simulink model "autopilot2e"  (R2017a)
settings: Solver=VariableStepAuto  StartTime=0.0  StopTime=300  RelTol=1e-3
values from neighbouring files (symbols this model uses):
  a_1 = 2.87    [auoschmilot.m]    (also in run_task_2f.m)
  a_2 = -0.65    [auoschmilot.m]    (also in run_task_2f.m)
  g = 9.81    [auoschmilot.m]    (also in run_task_2f.m)
  k_d_phi = (2*zeta_phi*w_n_phi-a_1)/a_2    [auoschmilot.m]    (also in run_task_2f.m)
  k_i_x = 0.195    [auoschmilot.m]    (also in run_task_2f.m)
  k_p_phi = -5/3    (= -1.66666666667)    [auoschmilot.m]    (also in run_task_2f.m)
  k_p_x = 2*zeta_X*w_n_x*V_g/g    [auoschmilot.m]    (also in run_task_2f.m)
  V_g = 637/3.6    (= 176.944444444)    [auoschmilot.m]    (also in run_task_2f.m)
settings Model: Creator=rokru  LastModifiedBy=emilal

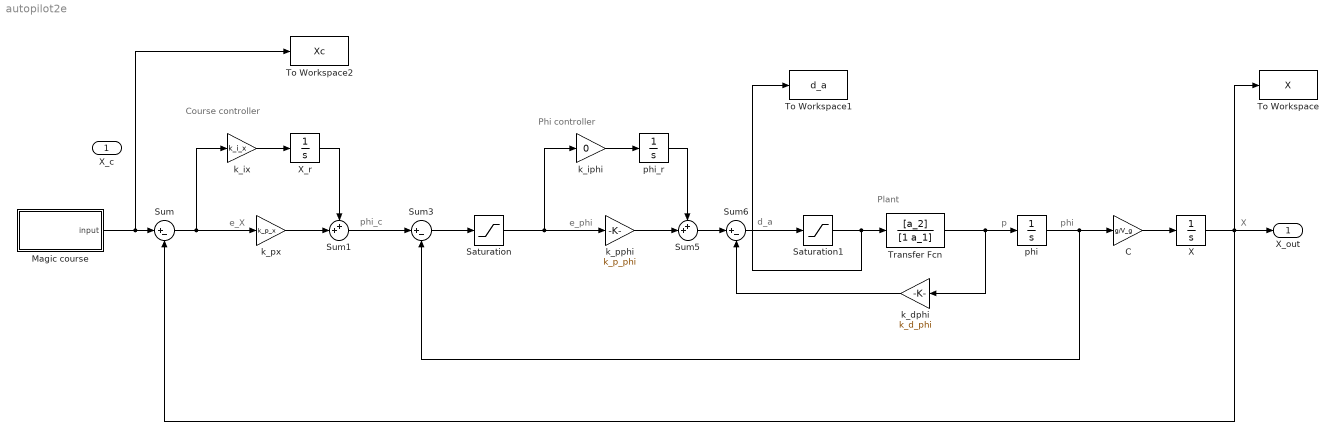
== system autopilot2e ==
  note: Course controller
  note: Phi controller
  note: Plant
  note: e_X
  note: e_phi
  note: phi_c
  note: X
  note: phi
  note: p
  note: d_a
  X_c : Inport
  C : Gain  Gain=g/V_g
  Magic course : Subsystem
  Saturation : Saturate  UpperLimit=25  LowerLimit=-25
  Saturation1 : Saturate  UpperLimit=15  LowerLimit=-15
  Sum : Sum  Inputs=|+-
  Sum1 : Sum  Inputs=++|
  Sum3 : Sum  Inputs=|+-
  Sum5 : Sum  Inputs=++|
  Sum6 : Sum  Inputs=|+-
  To Workspace : ToWorkspace  VariableName=X  SaveFormat=Timeseries  SampleTime=-1
  To Workspace1 : ToWorkspace  VariableName=d_a  SaveFormat=Timeseries  SampleTime=-1
  To Workspace2 : ToWorkspace  VariableName=Xc  SaveFormat=Timeseries  SampleTime=-1
  Transfer Fcn : TransferFcn  Numerator=[a_2]  Denominator=[1 a_1]
  X : Integrator
  X_r : Integrator
  k_dphi : Gain  Gain=k_d_phi
  k_iphi : Gain  Gain=0
  k_ix : Gain  Gain=k_i_x
  k_pphi : Gain  Gain=k_p_phi
  k_px : Gain  Gain=k_p_x
  phi : Integrator
  phi_r : Integrator
  X_out : Outport
  wires:
  Sum/1 -> k_px/1, k_ix/1
  k_ix/1 -> X_r/1
  X_r/1 -> Sum1/1
  Sum1/1 -> Sum3/1
  k_px/1 -> Sum1/2
  Sum5/1 -> Sum6/1
  k_pphi/1 -> Sum5/2
  Sum3/1 -> Saturation/1
  phi_r/1 -> Sum5/1
  k_iphi/1 -> phi_r/1
  Sum6/1 -> Saturation1/1
  Transfer Fcn/1 -> k_dphi/1, phi/1
  phi/1 -> C/1, Sum3/2
  k_dphi/1 -> Sum6/2
  X/1 -> To Workspace/1, Sum/2, X_out/1
  C/1 -> X/1
  Saturation/1 -> k_iphi/1, k_pphi/1
  Magic course/1(input) -> To Workspace2/1, Sum/1
  Saturation1/1 -> To Workspace1/1, Transfer Fcn/1

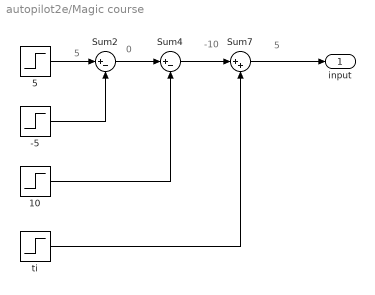
== system autopilot2e/Magic course ==
  note: 5
  note: -10
  note: 0
  note: 5
  -5 : Step  Time=100  After=5  SampleTime=0
  10 : Step  Time=150  After=10  SampleTime=0
  5 : Step  Time=10  After=5  SampleTime=0
  Sum2 : Sum  Inputs=|+-
  Sum4 : Sum  Inputs=|+-
  Sum7 : Sum  Inputs=|++
  ti : Step  Time=200  After=10  SampleTime=0
  input : Outport
  wires:
  10/1 -> Sum4/2
  ti/1 -> Sum7/2
  -5/1 -> Sum2/2
  Sum7/1 -> input/1
  5/1 -> Sum2/1
  Sum4/1 -> Sum7/1
  Sum2/1 -> Sum4/1
